simulink model "amon_model_2"  (R2025b)
settings: Solver=VariableStepAuto  StartTime=0.0  StopTime=dt  RelTol=1e-3
values from neighbouring files (symbols this model uses):
  EDF_max = 100    [amon_model.m]
  EDF_min = 0    [amon_model.m]
  g = [0; 0; 9.81]    [amon_model.m]
  servo1_offset = 0    [amon_model.m]
  servo2_offset = 0    [amon_model.m]
  servo3_offset = 0    [amon_model.m]
  servo4_offset = 0    [amon_model.m]
  servo_max = -45    [amon_model.m]
  servo_min = -45    [amon_model.m]
  tau_edf = 0    [amon_model.m]
  tau_servo = 0    [amon_model.m]
undefined symbols (not defined in the file or in its folder): k_x_minus, k_x_plus, k_y_minus, k_y_plus, n_x_minus, n_x_plus, n_y_minus, n_y_plus, r_x_minus, r_x_plus, r_y_minus, r_y_plus
libraries: aerolibconvert2 x4, simulink x1
settings Model: Creator=titit  LastModifiedBy=titit

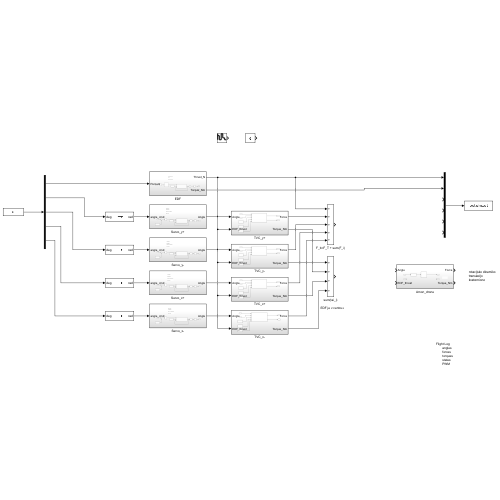
[thumbnail: Simulink's stored preview of the top-level diagram]
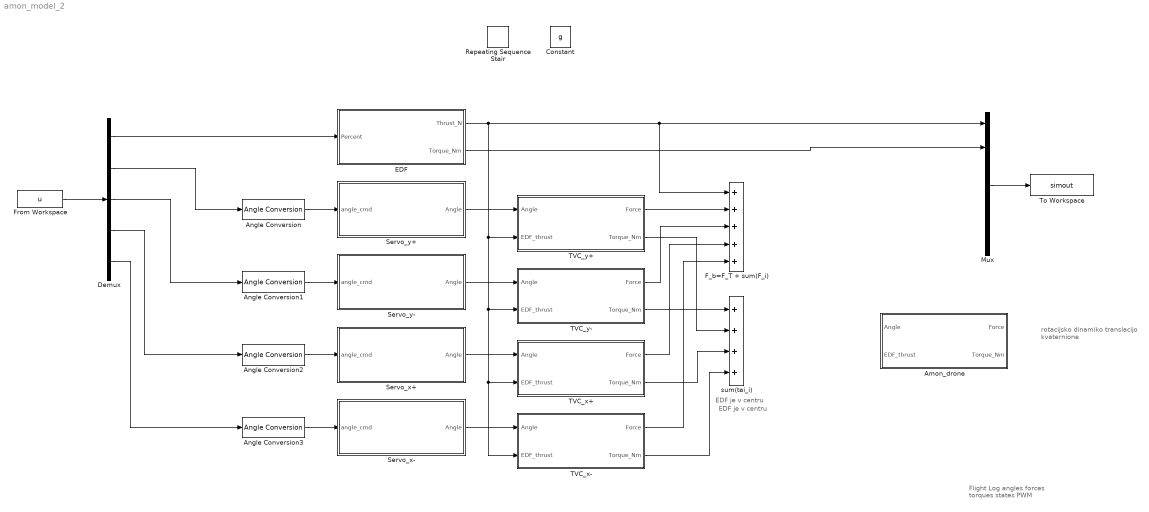
== system amon_model_2 ==
  note: EDF je v centru
  note: Flight Log
      | 	angles
      | 	forces
      | 	torques
      | 	states
      | 	PWM
  note: EDF je v centru
  note: rotacijsko dinamiko
      | translacijo
      | kvaternione
  Amon_drone : Subsystem
  Angle Conversion{,1..3} (4 alike) : aerolibconvert2/Angle Conversion  IU=deg  OU=rad
  Constant : Constant  Value=g
  Demux : Demux  Outputs=5
  EDF : Subsystem
  F_b=F_T + sum(F_i) : Sum  Inputs=+++++
  From Workspace : FromWorkspace  VariableName=u
  Mux : Mux  Inputs=6
  Repeating Sequence Stair : simulink/Sources/Repeating Sequence Stair  OutValues=[3 1 4 2 1].'  tsamp=-1  OutMin=[]  OutMax=[]  OutDataTypeStr=double  OutputDataTypeScalingMode=double  OutDataType=fixdt(0,8)  ConRadixGroup=Best Precision: Vector-wise  OutScaling=2^-12
  Servo_x+ : Subsystem
  Servo_x- : Subsystem
  Servo_y+ : Subsystem
  Servo_y- : Subsystem
  TVC_x+ : Subsystem
  TVC_x- : Subsystem
  TVC_y+ : Subsystem
  TVC_y- : Subsystem
  To Workspace : ToWorkspace  VariableName=simout  SaveFormat=Timeseries  SampleTime=-1
  sum(tai_i) : Sum  Inputs=++++
  wires:
  From Workspace/1 -> Demux/1
  Mux/1 -> To Workspace/1
  EDF/1(Thrust_N) -> TVC_y-/2(EDF_thrust), TVC_x-/2(EDF_thrust), TVC_x+/2(EDF_thrust), TVC_y+/2(EDF_thrust), F_b=F_T + sum(F_i)/1, Mux/1
  EDF/2(Torque_Nm) -> Mux/2
  Servo_y+/1(Angle) -> TVC_y+/1(Angle)
  Servo_y-/1(Angle) -> TVC_y-/1(Angle)
  Servo_x+/1(Angle) -> TVC_x+/1(Angle)
  Servo_x-/1(Angle) -> TVC_x-/1(Angle)
  Demux/1 -> EDF/1(Percent)
  Demux/2 -> Angle Conversion/1
  Demux/3 -> Angle Conversion1/1
  Demux/4 -> Angle Conversion2/1
  Demux/5 -> Angle Conversion3/1
  TVC_y+/1(Force) -> F_b=F_T + sum(F_i)/2
  TVC_y-/2(Torque_Nm) -> sum(tai_i)/1
  TVC_y+/2(Torque_Nm) -> sum(tai_i)/2
  TVC_y-/1(Force) -> F_b=F_T + sum(F_i)/3
  TVC_x+/1(Force) -> F_b=F_T + sum(F_i)/4
  TVC_x-/1(Force) -> F_b=F_T + sum(F_i)/5
  TVC_x+/2(Torque_Nm) -> sum(tai_i)/3
  TVC_x-/2(Torque_Nm) -> sum(tai_i)/4
  Angle Conversion/1 -> Servo_y+/1(angle_cmd)
  Angle Conversion1/1 -> Servo_y-/1(angle_cmd)
  Angle Conversion2/1 -> Servo_x+/1(angle_cmd)
  Angle Conversion3/1 -> Servo_x-/1(angle_cmd)

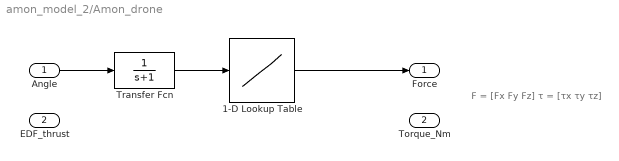
== system amon_model_2/Amon_drone ==
  note: F = [Fx Fy Fz]
      | τ = [τx τy τz]
  Angle : Inport
  EDF_thrust : Inport  Port=2
  1-D Lookup Table : Lookup_n-D  NumberOfTableDimensions=1  BreakpointsForDimension1=[-5:5]  Table=tanh([-5:5])  InternalRulePriority=Speed  RndMeth=Simplest
  Transfer Fcn : TransferFcn  Denominator=[1 1]
  Force : Outport
  Torque_Nm : Outport  Port=2
  wires:
  Transfer Fcn/1 -> 1-D Lookup Table/1
  Angle/1 -> Transfer Fcn/1
  1-D Lookup Table/1 -> Force/1

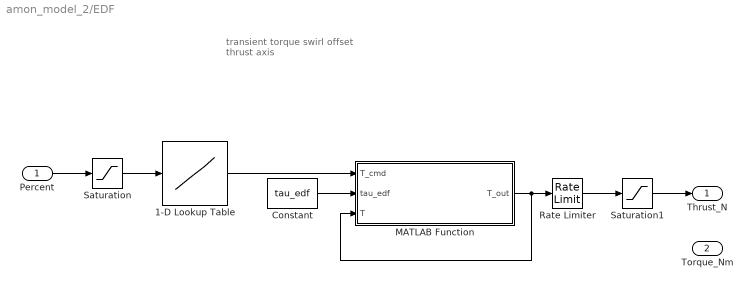
== system amon_model_2/EDF ==
  note: transient torque
      | swirl
      | offset thrust axis
  Percent : Inport
  1-D Lookup Table : Lookup_n-D  NumberOfTableDimensions=1  BreakpointsForDimension1=[-5:5]  Table=tanh([-5:5])  InternalRulePriority=Speed  RndMeth=Simplest
  Constant : Constant  Value=tau_edf
  MATLAB Function : MATLAB Function  TreatAsAtomicUnit=on
  Rate Limiter : RateLimiter  SampleTimeMode=inherited
  Saturation : Saturate  UpperLimit=EDF_max  LowerLimit=EDF_min
  Saturation1 : Saturate  UpperLimit=100  LowerLimit=0
  Thrust_N : Outport
  Torque_Nm : Outport  Port=2
  wires:
  Percent/1 -> Saturation/1
  Saturation1/1 -> Thrust_N/1
  1-D Lookup Table/1 -> MATLAB Function/1(T_cmd)
  MATLAB Function/1(T_out) -> MATLAB Function/3(T), Rate Limiter/1
  Saturation/1 -> 1-D Lookup Table/1
  Constant/1 -> MATLAB Function/2(tau_edf)
  Rate Limiter/1 -> Saturation1/1

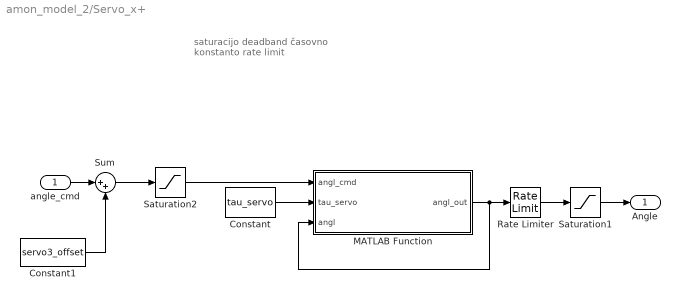
== system amon_model_2/Servo_x+ ==
  note: saturacijo
      | deadband
      | časovno konstanto
      | rate limit
  angle_cmd : Inport
  Constant : Constant  Value=tau_servo
  Constant1 : Constant  Value=servo3_offset
  MATLAB Function : MATLAB Function  TreatAsAtomicUnit=on
  Rate Limiter : RateLimiter  SampleTimeMode=inherited
  Saturation1 : Saturate  UpperLimit=servo_max  LowerLimit=servo_min
  Saturation2 : Saturate  UpperLimit=servo_max  LowerLimit=servo_min
  Sum : Sum  Inputs=|++
  Angle : Outport
  wires:
  Sum/1 -> Saturation2/1
  Constant/1 -> MATLAB Function/2(tau_servo)
  MATLAB Function/1(angl_out) -> Rate Limiter/1, MATLAB Function/3(angl)
  Saturation2/1 -> MATLAB Function/1(angl_cmd)
  Constant1/1 -> Sum/2
  angle_cmd/1 -> Sum/1
  Saturation1/1 -> Angle/1
  Rate Limiter/1 -> Saturation1/1

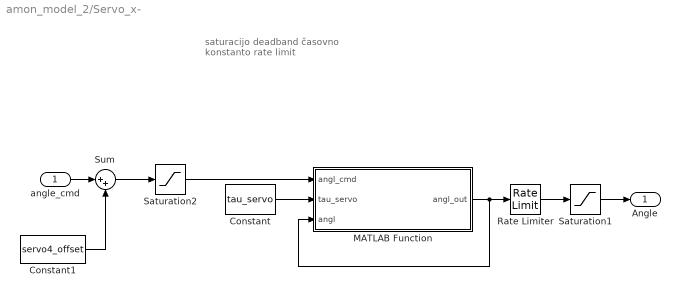
== system amon_model_2/Servo_x- ==
  note: saturacijo
      | deadband
      | časovno konstanto
      | rate limit
  angle_cmd : Inport
  Constant : Constant  Value=tau_servo
  Constant1 : Constant  Value=servo4_offset
  MATLAB Function : MATLAB Function  TreatAsAtomicUnit=on
  Rate Limiter : RateLimiter  SampleTimeMode=inherited
  Saturation1 : Saturate  UpperLimit=servo_max  LowerLimit=servo_min
  Saturation2 : Saturate  UpperLimit=servo_max  LowerLimit=servo_min
  Sum : Sum  Inputs=|++
  Angle : Outport
  wires:
  Constant/1 -> MATLAB Function/2(tau_servo)
  MATLAB Function/1(angl_out) -> Rate Limiter/1, MATLAB Function/3(angl)
  Saturation2/1 -> MATLAB Function/1(angl_cmd)
  Constant1/1 -> Sum/2
  angle_cmd/1 -> Sum/1
  Saturation1/1 -> Angle/1
  Rate Limiter/1 -> Saturation1/1
  Sum/1 -> Saturation2/1

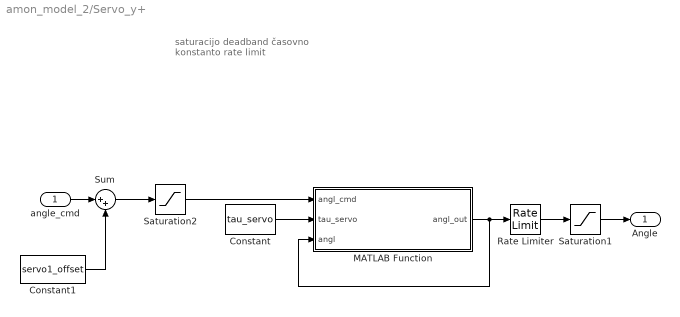
== system amon_model_2/Servo_y+ ==
  note: saturacijo
      | deadband
      | časovno konstanto
      | rate limit
  angle_cmd : Inport
  Constant : Constant  Value=tau_servo
  Constant1 : Constant  Value=servo1_offset
  MATLAB Function : MATLAB Function  TreatAsAtomicUnit=on
  Rate Limiter : RateLimiter  SampleTimeMode=inherited
  Saturation1 : Saturate  UpperLimit=servo_max  LowerLimit=servo_min
  Saturation2 : Saturate  UpperLimit=servo_max  LowerLimit=servo_min
  Sum : Sum  Inputs=|++
  Angle : Outport
  wires:
  Saturation2/1 -> MATLAB Function/1(angl_cmd)
  MATLAB Function/1(angl_out) -> MATLAB Function/3(angl), Rate Limiter/1
  Saturation1/1 -> Angle/1
  Constant/1 -> MATLAB Function/2(tau_servo)
  Rate Limiter/1 -> Saturation1/1
  angle_cmd/1 -> Sum/1
  Sum/1 -> Saturation2/1
  Constant1/1 -> Sum/2

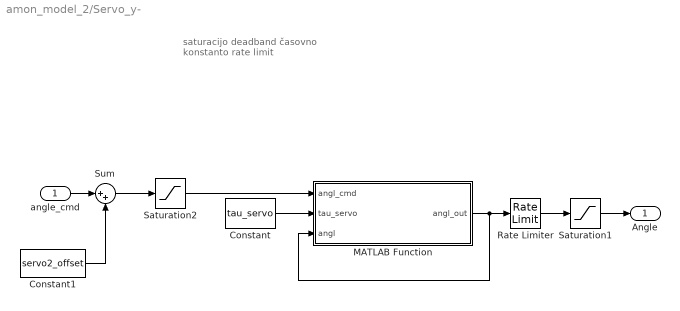
== system amon_model_2/Servo_y- ==
  note: saturacijo
      | deadband
      | časovno konstanto
      | rate limit
  angle_cmd : Inport
  Constant : Constant  Value=tau_servo
  Constant1 : Constant  Value=servo2_offset
  MATLAB Function : MATLAB Function  TreatAsAtomicUnit=on
  Rate Limiter : RateLimiter  SampleTimeMode=inherited
  Saturation1 : Saturate  UpperLimit=servo_max  LowerLimit=servo_min
  Saturation2 : Saturate  UpperLimit=servo_max  LowerLimit=servo_min
  Sum : Sum  Inputs=|++
  Angle : Outport
  wires:
  Sum/1 -> Saturation2/1
  Constant/1 -> MATLAB Function/2(tau_servo)
  MATLAB Function/1(angl_out) -> Rate Limiter/1, MATLAB Function/3(angl)
  Saturation2/1 -> MATLAB Function/1(angl_cmd)
  Constant1/1 -> Sum/2
  angle_cmd/1 -> Sum/1
  Saturation1/1 -> Angle/1
  Rate Limiter/1 -> Saturation1/1

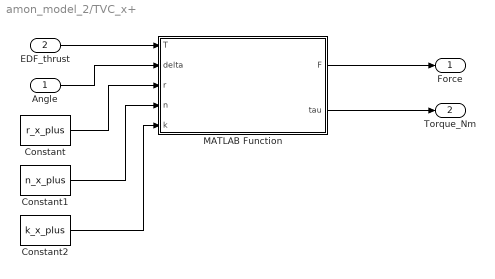
== system amon_model_2/TVC_x+ ==
  Angle : Inport
  EDF_thrust : Inport  Port=2
  Constant : Constant  Value=r_x_plus
  Constant1 : Constant  Value=n_x_plus
  Constant2 : Constant  Value=k_x_plus
  MATLAB Function : MATLAB Function  TreatAsAtomicUnit=on
  Force : Outport
  Torque_Nm : Outport  Port=2
  wires:
  Constant2/1 -> MATLAB Function/5(k)
  MATLAB Function/2(tau) -> Torque_Nm/1
  Constant1/1 -> MATLAB Function/4(n)
  EDF_thrust/1 -> MATLAB Function/1(T)
  MATLAB Function/1(F) -> Force/1
  Constant/1 -> MATLAB Function/3(r)
  Angle/1 -> MATLAB Function/2(delta)

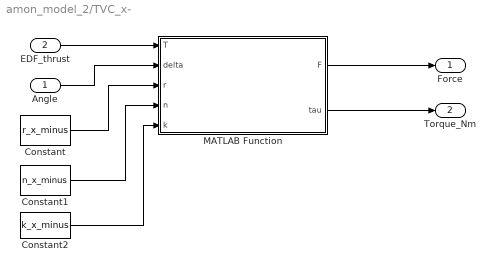
== system amon_model_2/TVC_x- ==
  Angle : Inport
  EDF_thrust : Inport  Port=2
  Constant : Constant  Value=r_x_minus
  Constant1 : Constant  Value=n_x_minus
  Constant2 : Constant  Value=k_x_minus
  MATLAB Function : MATLAB Function  TreatAsAtomicUnit=on
  Force : Outport
  Torque_Nm : Outport  Port=2
  wires:
  Constant2/1 -> MATLAB Function/5(k)
  MATLAB Function/2(tau) -> Torque_Nm/1
  Constant1/1 -> MATLAB Function/4(n)
  EDF_thrust/1 -> MATLAB Function/1(T)
  MATLAB Function/1(F) -> Force/1
  Constant/1 -> MATLAB Function/3(r)
  Angle/1 -> MATLAB Function/2(delta)

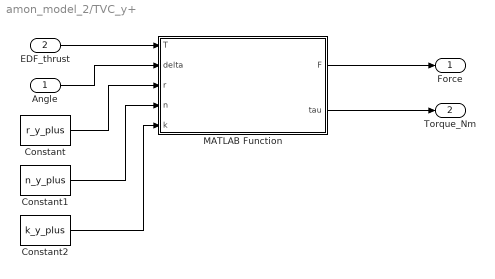
== system amon_model_2/TVC_y+ ==
  Angle : Inport
  EDF_thrust : Inport  Port=2
  Constant : Constant  Value=r_y_plus
  Constant1 : Constant  Value=n_y_plus
  Constant2 : Constant  Value=k_y_plus
  MATLAB Function : MATLAB Function  TreatAsAtomicUnit=on
  Force : Outport
  Torque_Nm : Outport  Port=2
  wires:
  EDF_thrust/1 -> MATLAB Function/1(T)
  Angle/1 -> MATLAB Function/2(delta)
  MATLAB Function/2(tau) -> Torque_Nm/1
  MATLAB Function/1(F) -> Force/1
  Constant/1 -> MATLAB Function/3(r)
  Constant1/1 -> MATLAB Function/4(n)
  Constant2/1 -> MATLAB Function/5(k)

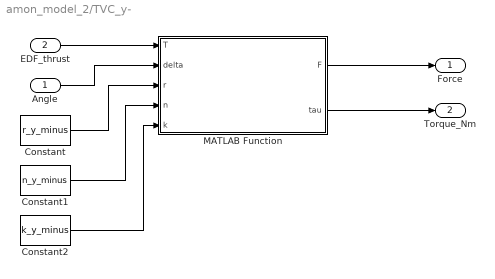
== system amon_model_2/TVC_y- ==
  Angle : Inport
  EDF_thrust : Inport  Port=2
  Constant : Constant  Value=r_y_minus
  Constant1 : Constant  Value=n_y_minus
  Constant2 : Constant  Value=k_y_minus
  MATLAB Function : MATLAB Function  TreatAsAtomicUnit=on
  Force : Outport
  Torque_Nm : Outport  Port=2
  wires:
  Constant2/1 -> MATLAB Function/5(k)
  MATLAB Function/2(tau) -> Torque_Nm/1
  Constant1/1 -> MATLAB Function/4(n)
  EDF_thrust/1 -> MATLAB Function/1(T)
  MATLAB Function/1(F) -> Force/1
  Constant/1 -> MATLAB Function/3(r)
  Angle/1 -> MATLAB Function/2(delta)

== matlab function amon_model_2/Servo_y+/MATLAB Function ==
  data: angl_cmd input; tau_servo input; angl_out output; angl input
function angl_out = servo_delay(angl_cmd, tau_servo, angl)
    angl_out = (1/tau_servo) * (angl_cmd - angl);
end

== matlab function amon_model_2/EDF/MATLAB Function ==
  data: T_cmd input; tau_edf input; T_out output; T input
function T_out = thrust_delay(T_cmd, tau_edf, T)
    T_out = (1/tau_edf) * (T_cmd - T);
end

== matlab function amon_model_2/Servo_y-/MATLAB Function ==
  data: angl_cmd input; tau_servo input; angl_out output; angl input
function angl_out = servo_delay(angl_cmd, tau_servo, angl)
    angl_out = (1/tau_servo) * (angl_cmd - angl);
end

== matlab function amon_model_2/Servo_x+/MATLAB Function ==
  data: angl_cmd input; tau_servo input; angl_out output; angl input
function angl_out = servo_delay(angl_cmd, tau_servo, angl)
    angl_out = (1/tau_servo) * (angl_cmd - angl);
end

== matlab function amon_model_2/Servo_x-/MATLAB Function ==
  data: angl_cmd input; tau_servo input; angl_out output; angl input
function angl_out = servo_delay(angl_cmd, tau_servo, angl)
    angl_out = (1/tau_servo) * (angl_cmd - angl);
end

== matlab function amon_model_2/TVC_y+/MATLAB Function ==
  data: T input; delta input; F output; r input; n input; k input; tau output
function [F, tau] = tvc_block(T, delta, r, n, k)
    F = T * k * delta * n; 
    tau = cross(r, F);
end

== matlab function amon_model_2/TVC_y-/MATLAB Function ==
  data: T input; delta input; F output; r input; n input; k input; tau output
function [F, tau] = tvc_block(T, delta, r, n, k)
    F = T * k * delta * n; 
    tau = cross(r, F);
end

== matlab function amon_model_2/TVC_x+/MATLAB Function ==
  data: T input; delta input; F output; r input; n input; k input; tau output
function [F, tau] = tvc_block(T, delta, r, n, k)
    F = T * k * delta * n; 
    tau = cross(r, F);
end

== matlab function amon_model_2/TVC_x-/MATLAB Function ==
  data: T input; delta input; F output; r input; n input; k input; tau output
function [F, tau] = tvc_block(T, delta, r, n, k)
    F = T * k * delta * n; 
    tau = cross(r, F);
end
